simulink model "Unity_6DOFMICO_Inversekine_v8"  (R2019b)
settings: Solver=ode5  StartTime=0.0  StopTime=inf  FixedStep=0.001  RelTol=1e-3
undefined symbols (not defined in the file): f, Sub02MIHM
libraries: instrumentlib x10, simulink x10, dspnetwork x6, powerlib_meascontrol x3, dspsrcs4 x1
(part 1 of 3)
settings Model: Creator=nisit  LastModifiedBy=e295q643

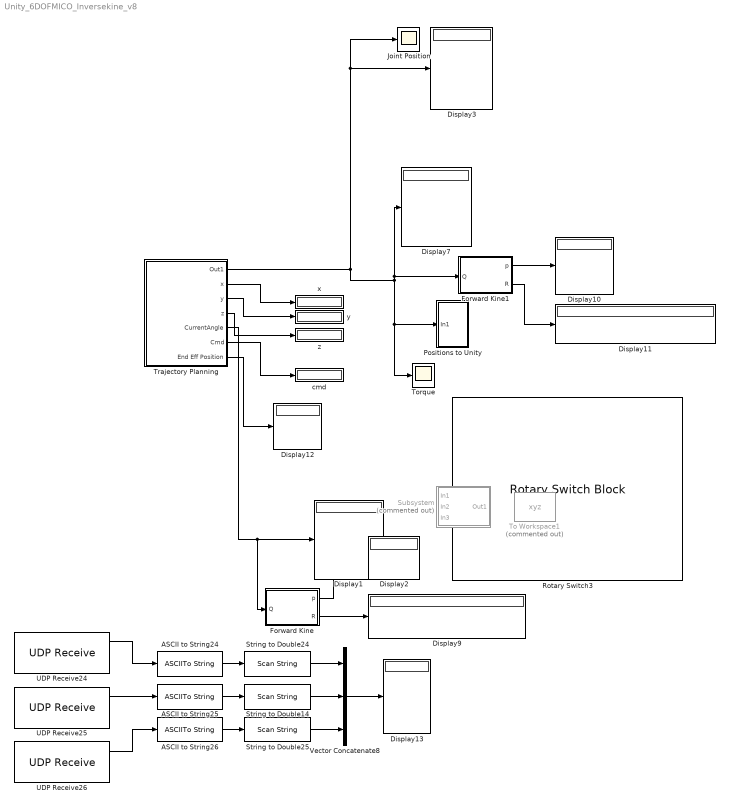
== system Unity_6DOFMICO_Inversekine_v8 ==
  ASCII to String24 : ASCIIToString
  ASCII to String25 : ASCIIToString
  ASCII to String26 : ASCIIToString
  Display{1..3,7,9..13} (9 alike) : Display
  Forward Kine : MATLAB Function  TreatAsAtomicUnit=on
  Forward Kine1 : MATLAB Function  TreatAsAtomicUnit=on
  Joint Position : Scope
  Positions to Unity : Subsystem
  Rotary Switch3 : RotarySwitchBlock
      settings: Values={{'Left', 'Right', 'Up', 'Down', 'In', 'Out', 'Resting', 'Reset'}, [1 2 3 4 5 6 7 8]}
  String to Double14 : ScanString  Format="\"%lf\""
  String to Double24 : ScanString  Format="\"%lf\""
  String to Double25 : ScanString  Format="\"%lf\""
  Subsystem : Subsystem  Commented=on
  To Workspace1 : ToWorkspace  Commented=on  VariableName=xyz  SampleTime=-1
      settings: Save2DSignal=2-D array (concatenate along first dimension)
  Torque : Scope
  Trajectory Planning : Subsystem
  UDP Receive24 : instrumentlib/UDP Receive  Host=localhost  Port=5100  LocalPort=5100  EnablePortSharing=off  GetLatestData=off  DataSize="[5  1]"  DataType=uint8  ASCIIFormatting=%f,  Terminator=LF  ByteOrder=BigEndian  EnableBlockingMode=off  Timeout=10  SampleTime=0.01  LocalAddress=127.0.0.1
  UDP Receive25 : instrumentlib/UDP Receive  Host=localhost  Port=5200  LocalPort=5200  EnablePortSharing=off  GetLatestData=off  DataSize="[5  1]"  DataType=uint8  ASCIIFormatting=%f,  Terminator=LF  ByteOrder=BigEndian  EnableBlockingMode=off  Timeout=10  SampleTime=0.01  LocalAddress=127.0.0.1
  UDP Receive26 : instrumentlib/UDP Receive  Host=localhost  Port=5300  LocalPort=5300  EnablePortSharing=off  GetLatestData=off  DataSize="[5  1]"  DataType=uint8  ASCIIFormatting=%f,  Terminator=LF  ByteOrder=BigEndian  EnableBlockingMode=off  Timeout=10  SampleTime=0.01  LocalAddress=127.0.0.1
  Vector Concatenate8 : Concatenate  NumInputs=3
  cmd : Display
  x : Display
  y : Display
  z : Display
  wires:
  Trajectory Planning/2(x) -> x/1
  Trajectory Planning/3(y) -> y/1
  Trajectory Planning/4(z) -> z/1
  Trajectory Planning/5("CurrentAngle ") -> Display1/1, Forward Kine/1(Q)
  Forward Kine/1(p) -> Display2/1
  Forward Kine/2(R) -> Display9/1
  Forward Kine1/2(R) -> Display11/1
  Forward Kine1/1(p) -> Display10/1
  Trajectory Planning/1(Out1) -> Display7/1, Forward Kine1/1(Q), Torque/1, Positions to Unity/1(In1), Display3/1, Joint Position/1
  Trajectory Planning/6(Cmd) -> cmd/1
  Subsystem/1(Out1) -> To Workspace1/1
  Trajectory Planning/7(End Eff Position) -> Display12/1
  Vector Concatenate8/1 -> Display13/1
  UDP Receive24/1 -> ASCII to String24/1
  String to Double24/1 -> Vector Concatenate8/1
  ASCII to String26/1 -> String to Double25/1
  UDP Receive25/1 -> ASCII to String25/1
  UDP Receive26/1 -> ASCII to String26/1
  String to Double25/1 -> Vector Concatenate8/3
  String to Double14/1 -> Vector Concatenate8/2
  ASCII to String24/1 -> String to Double24/1
  ASCII to String25/1 -> String to Double14/1

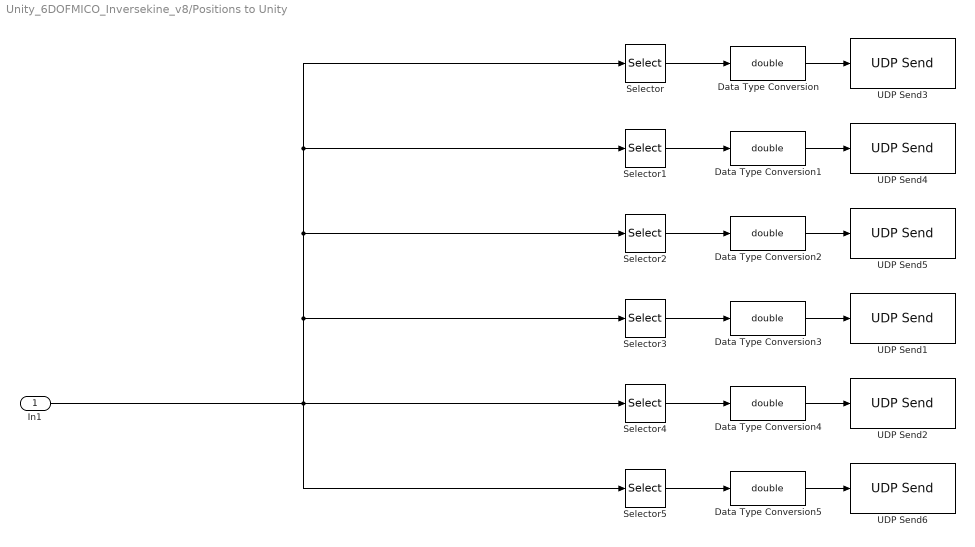
== system Unity_6DOFMICO_Inversekine_v8/Positions to Unity ==
  In1 : Inport
  Data Type Conversion{,1..5} (6 alike) : DataTypeConversion  OutDataTypeStr=double  ConvertRealWorld=Stored Integer (SI)
  Selector : Selector  InputPortWidth=6  IndexOptions=Index vector (dialog)  Indices=[1]  OutputSizes=1
  Selector1 : Selector  InputPortWidth=6  IndexOptions=Index vector (dialog)  Indices=[2]  OutputSizes=1
  Selector2 : Selector  InputPortWidth=6  IndexOptions=Index vector (dialog)  Indices=[3]  OutputSizes=1
  Selector3 : Selector  InputPortWidth=6  IndexOptions=Index vector (dialog)  Indices=[4]  OutputSizes=1
  Selector4 : Selector  InputPortWidth=6  IndexOptions=Index vector (dialog)  Indices=[5]  OutputSizes=1
  Selector5 : Selector  InputPortWidth=6  IndexOptions=Index vector (dialog)  Indices=[6]  OutputSizes=1
  UDP Send1 : dspnetwork/UDP Send  remoteURL='127.0.0.1'  remotePort=3004  localURL='0.0.0.0'  localPortSource=Automatically determine  localPort=-1  sampletime=-1  blockPlatform=[]  separateLengthPort=0
  UDP Send2 : dspnetwork/UDP Send  remoteURL='127.0.0.1'  remotePort=3005  localURL='0.0.0.0'  localPortSource=Automatically determine  localPort=-1  sampletime=-1  blockPlatform=[]  separateLengthPort=0
  UDP Send3 : dspnetwork/UDP Send  remoteURL='127.0.0.1'  remotePort=3001  localURL='0.0.0.0'  localPortSource=Automatically determine  localPort=-1  sampletime=-1  blockPlatform=[]  separateLengthPort=0
  UDP Send4 : dspnetwork/UDP Send  remoteURL='127.0.0.1'  remotePort=3002  localURL='0.0.0.0'  localPortSource=Automatically determine  localPort=-1  sampletime=-1  blockPlatform=[]  separateLengthPort=0
  UDP Send5 : dspnetwork/UDP Send  remoteURL='127.0.0.1'  remotePort=3003  localURL='0.0.0.0'  localPortSource=Automatically determine  localPort=-1  sampletime=-1  blockPlatform=[]  separateLengthPort=0
  UDP Send6 : dspnetwork/UDP Send  remoteURL='127.0.0.1'  remotePort=3006  localURL='0.0.0.0'  localPortSource=Automatically determine  localPort=-1  sampletime=-1  blockPlatform=[]  separateLengthPort=0
  wires:
  Data Type Conversion2/1 -> UDP Send5/1
  Selector5/1 -> Data Type Conversion5/1
  In1/1 -> Selector/1, Selector1/1, Selector2/1, Selector3/1, Selector5/1, Selector4/1
  Selector2/1 -> Data Type Conversion2/1
  Data Type Conversion3/1 -> UDP Send1/1
  Data Type Conversion1/1 -> UDP Send4/1
  Data Type Conversion5/1 -> UDP Send6/1
  Selector1/1 -> Data Type Conversion1/1
  Selector4/1 -> Data Type Conversion4/1
  Selector3/1 -> Data Type Conversion3/1
  Data Type Conversion4/1 -> UDP Send2/1
  Selector/1 -> Data Type Conversion/1
  Data Type Conversion/1 -> UDP Send3/1

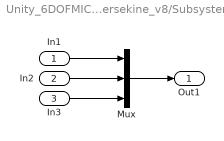
== system Unity_6DOFMICO_Inversekine_v8/Subsystem ==
  In1 : Inport
  In2 : Inport  Port=2
  In3 : Inport  Port=3
  Mux : Mux  Inputs=3
  Out1 : Outport
  wires:
  In1/1 -> Mux/1
  In2/1 -> Mux/2
  Mux/1 -> Out1/1
  In3/1 -> Mux/3

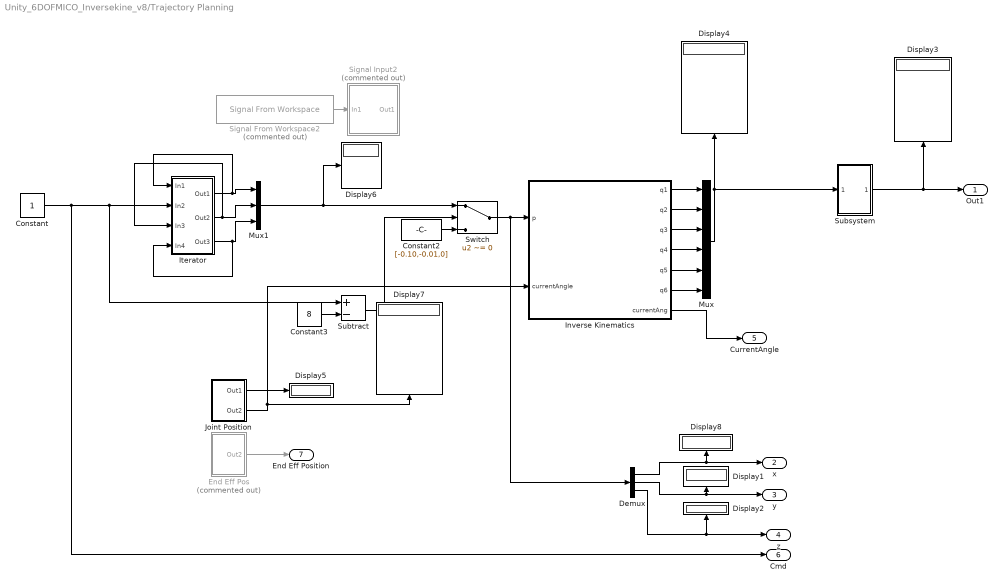
== system Unity_6DOFMICO_Inversekine_v8/Trajectory Planning ==
  Constant : Constant
  Constant2 : Constant  Value=[-0.10,-0.01,0]
  Constant3 : Constant  Value=8
  Demux : Demux  Outputs=3
  Display{1..8} (8 alike) : Display
  End Eff Pos : Subsystem  Commented=on
  Inverse Kinematics : MATLAB Function  TreatAsAtomicUnit=on
  Iterator : Subsystem
  Joint Position : Subsystem
  Mux : Mux  Inputs=6
      settings: DisplayOption=signals
  Mux1 : Mux  Inputs=3
  Signal From Workspace2 : dspsrcs4/Signal From Workspace  Commented=on  X=transpose(Sub02MIHM)  Ts=0.004  nsamps=1  OutputAfterFinalValue=Setting to zero  ignoreOrWarnInputAndFrameLengths=off  OutputFrames=off
  Signal Input2 : Subsystem  Commented=on
  Subsystem : Subsystem
  Subtract : Sum  Inputs=+-
  Switch : Switch  Criteria=u2 ~= 0
  Out1 : Outport
  x : Outport  Port=2
  y : Outport  Port=3
  z : Outport  Port=4
  "CurrentAngle " : Outport  Port=5
  Cmd : Outport  Port=6
  End Eff Position : Outport  Port=7
  wires:
  Iterator/2(Out2) -> Mux1/2, Iterator/3(In3)
  Iterator/1(Out1) -> Mux1/1, Iterator/1(In1)
  Inverse Kinematics/2(q2) -> Mux/2
  Iterator/3(Out3) -> Mux1/3, Iterator/4(In4)
  Inverse Kinematics/6(q6) -> Mux/6
  Inverse Kinematics/4(q4) -> Mux/4
  Inverse Kinematics/1(q1) -> Mux/1
  Inverse Kinematics/3(q3) -> Mux/3
  Signal From Workspace2/1 -> Signal Input2/1(In1)
  Mux/1 -> Subsystem/1(In1), Display4/1
  Inverse Kinematics/5(q5) -> Mux/5
  Subsystem/1(Out1) -> Out1/1, Display3/1
  Joint Position/1(Out1) -> Display5/1
  Joint Position/2(Out2) -> Display7/1, Inverse Kinematics/2(currentAngle)
  Demux/1 -> Display8/1, x/1
  Demux/2 -> Display1/1, y/1
  Demux/3 -> Display2/1, z/1
  Mux1/1 -> Display6/1, Switch/1
  Subtract/1 -> Switch/2
  Constant2/1 -> Switch/3
  Constant3/1 -> Subtract/2
  Constant/1 -> Cmd/1, Subtract/1, Iterator/2(In2)
  Switch/1 -> Demux/1, Inverse Kinematics/1(p)
  Inverse Kinematics/7(currentAng) -> "CurrentAngle "/1
  End Eff Pos/1(Out2) -> End Eff Position/1

== system Unity_6DOFMICO_Inversekine_v8/Trajectory Planning/End Eff Pos ==
  ASCII to String : ASCIIToString
  Display : Display
  String to Double : ScanString  Format="\"%lf\""
  UDP Receive : instrumentlib/UDP Receive  Host=localhost  Port=5000  LocalPort=5000  EnablePortSharing=off  GetLatestData=off  DataSize="[3  1]"  DataType=uint8  ASCIIFormatting=%f,  Terminator=LF  ByteOrder=BigEndian  EnableBlockingMode=off  Timeout=10  SampleTime=0.01  LocalAddress=127.0.0.1
  Out2 : Outport
  wires:
  UDP Receive/2 -> Display/1
  ASCII to String/1 -> String to Double/1
  UDP Receive/1 -> ASCII to String/1
  String to Double/1 -> Out2/1

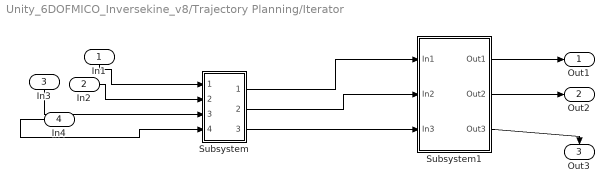
== system Unity_6DOFMICO_Inversekine_v8/Trajectory Planning/Iterator ==
  In1 : Inport
  In2 : Inport  Port=2
  In3 : Inport  Port=3
  In4 : Inport  Port=4
  Subsystem : Subsystem
  Subsystem1 : Subsystem  VariantControlMode=Label  Variant=on  VariantControl=Variant1  LabelModeActiveChoice=Variant1
  Out1 : Outport
  Out2 : Outport  Port=2
  Out3 : Outport  Port=3
  wires:
  In1/1 -> Subsystem/1(In1)
  In3/1 -> Subsystem/3(In3)
  In4/1 -> Subsystem/4(In4)
  In2/1 -> Subsystem/2(In2)
  Subsystem/1(Out1) -> Subsystem1/1("In1 ")
  Subsystem/2(Out2) -> Subsystem1/2("In2 ")
  Subsystem/3(Out3) -> Subsystem1/3("In3 ")
  Subsystem1/1(" Out1") -> Out1/1
  Subsystem1/2(" Out2") -> Out2/1
  Subsystem1/3(" Out3") -> Out3/1

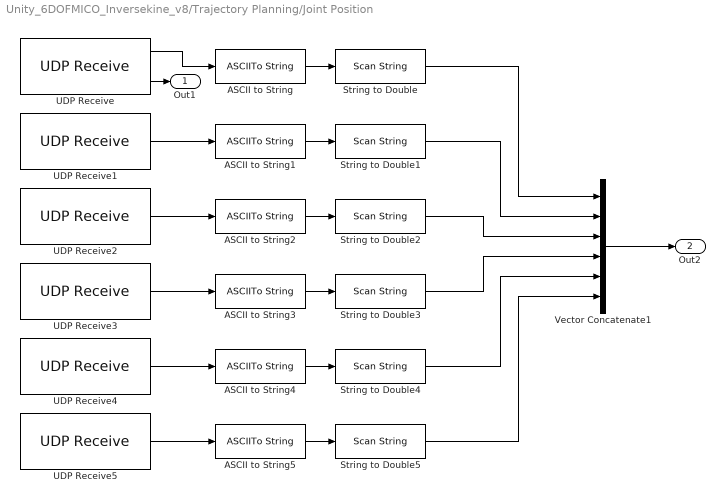
== system Unity_6DOFMICO_Inversekine_v8/Trajectory Planning/Joint Position ==
  ASCII to String{,1..5} (6 alike) : ASCIIToString
  String to Double{,1..5} (6 alike) : ScanString  Format="\"%lf\""
  UDP Receive : instrumentlib/UDP Receive  Host=localhost  Port=2001  LocalPort=2001  EnablePortSharing=off  GetLatestData=off  DataSize="[5  1]"  DataType=uint8  ASCIIFormatting=%f,  Terminator=LF  ByteOrder=BigEndian  EnableBlockingMode=off  Timeout=10  SampleTime=0.01  LocalAddress=127.0.0.1
  UDP Receive1 : instrumentlib/UDP Receive  Host=localhost  Port=2002  LocalPort=2002  EnablePortSharing=off  GetLatestData=off  DataSize="[5  1]"  DataType=uint8  ASCIIFormatting=%f,  Terminator=LF  ByteOrder=BigEndian  EnableBlockingMode=on  Timeout=10  SampleTime=0.01  LocalAddress=127.0.0.1
  UDP Receive2 : instrumentlib/UDP Receive  Host=localhost  Port=2003  LocalPort=2003  EnablePortSharing=off  GetLatestData=off  DataSize="[5  1]"  DataType=uint8  ASCIIFormatting=%f,  Terminator=LF  ByteOrder=BigEndian  EnableBlockingMode=on  Timeout=10  SampleTime=0.01  LocalAddress=127.0.0.1
  UDP Receive3 : instrumentlib/UDP Receive  Host=localhost  Port=2004  LocalPort=2004  EnablePortSharing=off  GetLatestData=off  DataSize="[5  1]"  DataType=uint8  ASCIIFormatting=%f,  Terminator=LF  ByteOrder=BigEndian  EnableBlockingMode=on  Timeout=10  SampleTime=0.01  LocalAddress=127.0.0.1
  UDP Receive4 : instrumentlib/UDP Receive  Host=localhost  Port=2005  LocalPort=2005  EnablePortSharing=off  GetLatestData=off  DataSize="[5  1]"  DataType=uint8  ASCIIFormatting=%f,  Terminator=LF  ByteOrder=BigEndian  EnableBlockingMode=on  Timeout=10  SampleTime=0.01  LocalAddress=127.0.0.1
  UDP Receive5 : instrumentlib/UDP Receive  Host=localhost  Port=2006  LocalPort=2006  EnablePortSharing=off  GetLatestData=off  DataSize="[5  1]"  DataType=uint8  ASCIIFormatting=%f,  Terminator=LF  ByteOrder=BigEndian  EnableBlockingMode=on  Timeout=10  SampleTime=0.01  LocalAddress=127.0.0.1
  Vector Concatenate1 : Concatenate  NumInputs=6
  Out1 : Outport
  Out2 : Outport  Port=2
  wires:
  String to Double3/1 -> Vector Concatenate1/4
  String to Double4/1 -> Vector Concatenate1/5
  UDP Receive1/1 -> ASCII to String1/1
  String to Double1/1 -> Vector Concatenate1/2
  UDP Receive4/1 -> ASCII to String4/1
  UDP Receive3/1 -> ASCII to String3/1
  String to Double/1 -> Vector Concatenate1/1
  ASCII to String4/1 -> String to Double4/1
  String to Double2/1 -> Vector Concatenate1/3
  ASCII to String2/1 -> String to Double2/1
  ASCII to String3/1 -> String to Double3/1
  Vector Concatenate1/1 -> Out2/1
  String to Double5/1 -> Vector Concatenate1/6
  ASCII to String1/1 -> String to Double1/1
  UDP Receive/1 -> ASCII to String/1
  UDP Receive5/1 -> ASCII to String5/1
  UDP Receive2/1 -> ASCII to String2/1
  ASCII to String5/1 -> String to Double5/1
  ASCII to String/1 -> String to Double/1
  UDP Receive/2 -> Out1/1

== system Unity_6DOFMICO_Inversekine_v8/Trajectory Planning/Signal Input2 ==
  In1 : Inport
  Iterator Input : Subsystem
  Subsystem1 : Subsystem
  Out1 : Outport
  wires:
  Subsystem1/1(Out1) -> Iterator Input/1(In1)
  Subsystem1/3(Out3) -> Iterator Input/3(In3)
  In1/1 -> Subsystem1/1(In1)
  Subsystem1/4(Out4) -> Iterator Input/4(In4)
  Subsystem1/7(Out7) -> Iterator Input/7(In7)
  Subsystem1/2(Out2) -> Iterator Input/2(In2)
  Subsystem1/6(Out6) -> Iterator Input/6(In6)
  Subsystem1/5(Out5) -> Iterator Input/5(In5)
  Iterator Input/1(Out1) -> Out1/1

== system Unity_6DOFMICO_Inversekine_v8/Trajectory Planning/Subsystem ==
  In1 : Inport
  Demux : Demux  Outputs=6
  Mux1 : Mux  Inputs=6
  Out1 : Outport
  wires:
  Demux/2 -> Mux1/2
  Demux/5 -> Mux1/5
  Demux/1 -> Mux1/1
  Mux1/1 -> Out1/1
  Demux/6 -> Mux1/6
  In1/1 -> Demux/1
  Demux/4 -> Mux1/4
  Demux/3 -> Mux1/3

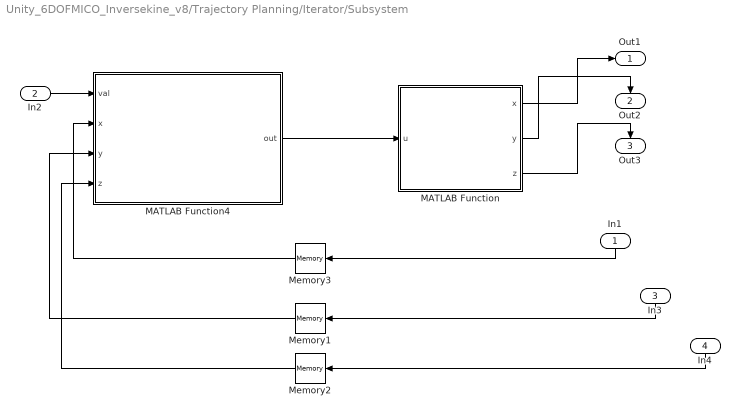
== system Unity_6DOFMICO_Inversekine_v8/Trajectory Planning/Iterator/Subsystem ==
  In1 : Inport
  In2 : Inport  Port=2
  In3 : Inport  Port=3
  In4 : Inport  Port=4
  MATLAB Function : MATLAB Function  TreatAsAtomicUnit=on
  MATLAB Function4 : MATLAB Function  TreatAsAtomicUnit=on
  Memory1 : Memory
  Memory2 : Memory
  Memory3 : Memory
  Out1 : Outport
  Out2 : Outport  Port=2
  Out3 : Outport  Port=3
  wires:
  In2/1 -> MATLAB Function4/1(val)
  MATLAB Function/2(y) -> Out2/1
  MATLAB Function/3(z) -> Out3/1
  MATLAB Function/1(x) -> Out1/1
  MATLAB Function4/1(out) -> MATLAB Function/1(u)
  In1/1 -> Memory3/1
  In3/1 -> Memory1/1
  In4/1 -> Memory2/1
  Memory3/1 -> MATLAB Function4/2(x)
  Memory1/1 -> MATLAB Function4/3(y)
  Memory2/1 -> MATLAB Function4/4(z)

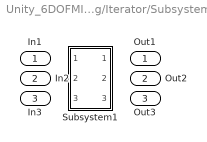
== system Unity_6DOFMICO_Inversekine_v8/Trajectory Planning/Iterator/Subsystem1 ==
  "In1 " : Inport
  "In2 " : Inport  Port=2
  "In3 " : Inport  Port=3
  Subsystem1 : Subsystem  VariantControl=Variant1
  " Out1" : Outport
  " Out2" : Outport  Port=2
  " Out3" : Outport  Port=3

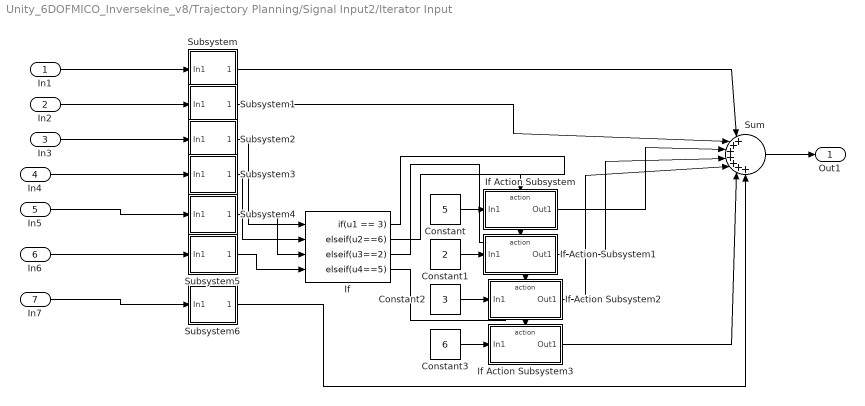
== system Unity_6DOFMICO_Inversekine_v8/Trajectory Planning/Signal Input2/Iterator Input ==
  In1 : Inport
  In2 : Inport  Port=2
  In3 : Inport  Port=3
  In4 : Inport  Port=4
  In5 : Inport  Port=5
  In6 : Inport  Port=6
  In7 : Inport  Port=7
  Constant : Constant  Value=5
  Constant1 : Constant  Value=2
  Constant2 : Constant  Value=3
  Constant3 : Constant  Value=6
  If : If  NumInputs=4  IfExpression=u1 == 3  ElseIfExpressions=u2==6,u3==2,u4==5  ShowElse=off
  If Action Subsystem : Subsystem  TreatAsAtomicUnit=on
  If Action Subsystem1 : Subsystem  TreatAsAtomicUnit=on
  If Action Subsystem2 : Subsystem  TreatAsAtomicUnit=on
  If Action Subsystem3 : Subsystem  TreatAsAtomicUnit=on
  Subsystem : Subsystem
  Subsystem1 : Subsystem
  Subsystem2 : Subsystem
  Subsystem3 : Subsystem
  Subsystem4 : Subsystem
  Subsystem5 : Subsystem
  Subsystem6 : Subsystem
  Sum : Sum  Inputs=|+++++++
  Out1 : Outport
  wires:
  Sum/1 -> Out1/1
  In5/1 -> Subsystem4/1(In1)
  In2/1 -> Subsystem1/1(In1)
  Subsystem/1(Out1) -> Sum/1
  In4/1 -> Subsystem3/1(In1)
  Subsystem1/1(Out1) -> Sum/2
  In1/1 -> Subsystem/1(In1)
  In3/1 -> Subsystem2/1(In1)
  In6/1 -> Subsystem5/1(In1)
  In7/1 -> Subsystem6/1(In1)
  If/1 -> If Action Subsystem/Action
  Constant/1 -> If Action Subsystem/1(In1)
  If/2 -> If Action Subsystem1/Action
  If/3 -> If Action Subsystem2/Action
  If/4 -> If Action Subsystem3/Action
  Constant2/1 -> If Action Subsystem2/1(In1)
  Constant1/1 -> If Action Subsystem1/1(In1)
  Constant3/1 -> If Action Subsystem3/1(In1)
  Subsystem2/1(Out1) -> If/1
  Subsystem3/1(Out1) -> If/2
  Subsystem4/1(Out1) -> If/3
  Subsystem5/1(Out1) -> If/4
  Subsystem6/1(Out1) -> Sum/7
  If Action Subsystem/1(Out1) -> Sum/3
  If Action Subsystem1/1(Out1) -> Sum/4
  If Action Subsystem2/1(Out1) -> Sum/5
  If Action Subsystem3/1(Out1) -> Sum/6

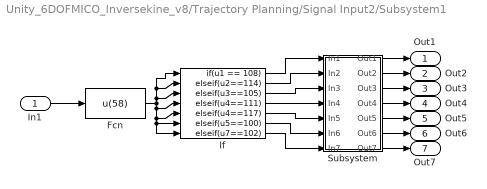
== system Unity_6DOFMICO_Inversekine_v8/Trajectory Planning/Signal Input2/Subsystem1 ==
  In1 : Inport
  Fcn : Fcn  Expr=u(58)
  If : If  NumInputs=7  IfExpression=u1 == 108  ElseIfExpressions=u2==114,u3==105,u4==111,u4==117,u5==100,u7==102  ShowElse=off
  Subsystem : Subsystem
  Out1 : Outport
  Out2 : Outport  Port=2
  Out3 : Outport  Port=3
  Out4 : Outport  Port=4
  Out5 : Outport  Port=5
  Out6 : Outport  Port=6
  Out7 : Outport  Port=7
  wires:
  If/6 -> Subsystem/6(In6)
  If/2 -> Subsystem/2(In2)
  If/4 -> Subsystem/4(In4)
  If/7 -> Subsystem/7(In7)
  If/3 -> Subsystem/3(In3)
  Fcn/1 -> If/1, If/2, If/3, If/7, If/6, If/5, If/4
  If/1 -> Subsystem/1(In1)
  If/5 -> Subsystem/5(In5)
  Subsystem/1(Out1) -> Out1/1
  Subsystem/2(Out2) -> Out2/1
  Subsystem/3(Out3) -> Out3/1
  In1/1 -> Fcn/1
  Subsystem/6(Out6) -> Out6/1
  Subsystem/5(Out5) -> Out5/1
  Subsystem/4(Out4) -> Out4/1
  Subsystem/7(Out7) -> Out7/1

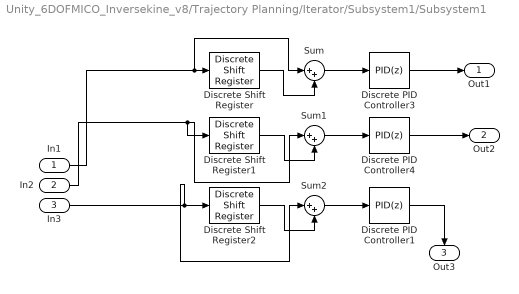
== system Unity_6DOFMICO_Inversekine_v8/Trajectory Planning/Iterator/Subsystem1/Subsystem1 ==
  In1 : Inport
  In2 : Inport  Port=2
  In3 : Inport  Port=3
  Discrete Shift Register : powerlib_meascontrol/Additional Components/Discrete Shift Register  NSamples=1  InitialValue=0  Ts=-1
      settings: SourceProductName=Simscape Electrical  SourceProductBaseCode=PS
  Discrete Shift Register1 : powerlib_meascontrol/Additional Components/Discrete Shift Register  NSamples=1  InitialValue=0  Ts=-1
      settings: SourceProductName=Simscape Electrical  SourceProductBaseCode=PS
  Discrete Shift Register2 : powerlib_meascontrol/Additional Components/Discrete Shift Register  NSamples=1  InitialValue=0  Ts=-1
      settings: SourceProductName=Simscape Electrical  SourceProductBaseCode=PS
  Discrete PID Controller1 : simulink/Continuous/PID Controller  Controller=PID  Form=Parallel  TimeDomain=Discrete-time  SampleTime=-1  IntegratorMethod=Forward Euler  FilterMethod=Forward Euler  ControllerParametersSource=internal  P=1  I=1  D=0  UseFilter=on  N=100  TunerSelectOption=Transfer Function Based (PID Tuner App)  InitialConditionSource=internal  InitialConditionForIntegrator=0  InitialConditionForFilter=0  DifferentiatorICPrevScaledInput=0  ExternalReset=none  TrackingMode=off  Kt=1  LimitOutput=off  UpperSaturationLimit=inf  LowerSaturationLimit=-inf  LinearizeAsGain=off  AntiWindupMode=none  Kb=1  POutMin=[]  POutMax=[]  IOutMin=[]  IOutMax=[]  DOutMin=[]  DOutMax=[]  NOutMin=[]  NOutMax=[]  SumOutMin=[]  SumOutMax=[]  SaturationOutMin=[]  SaturationOutMax=[]  PParamMin=[]  PParamMax=[]  IParamMin=[]  IParamMax=[]  DParamMin=[]  DParamMax=[]  NParamMin=[]  NParamMax=[]  KbParamMin=[]  KbParamMax=[]  KtParamMin=[]  KtParamMax=[]  KbOutMin=[]  KbOutMax=[]  KtOutMin=[]  KtOutMax=[]  IntegratorOutMin=[]  IntegratorOutMax=[]  FilterOutMin=[]  FilterOutMax=[]  SumI1OutMin=[]  SumI1OutMax=[]  SumI2OutMin=[]  SumI2OutMax=[]  SumI3OutMin=[]  SumI3OutMax=[]  SumI4OutMin=[]  SumI4OutMax=[]  SumDOutMin=[]  SumDOutMax=[]  DifferentiatorOutMin=[]  DifferentiatorOutMax=[]  FilterDiffOutCoefMin=[]  FilterDiffOutCoefMax=[]  ReciprocalOutMin=[]  ReciprocalOutMax=[]  SumDenOutMin=[]  SumDenOutMax=[]  SumNumOutMin=[]  SumNumOutMax=[]  DivideOutMin=[]  DivideOutMax=[]  IntegratorContinuousStateAttributes=''  IntegratorStateMustResolveToSignalObject=off  IntegratorRTWStateStorageClass=Auto  FilterContinuousStateAttributes=''  FilterStateMustResolveToSignalObject=off  FilterRTWStateStorageClass=Auto  ParallelPVariant=InternalParameters  IdealPVariant=Disabled  IVariant=InternalParameters  DVariant=InternalParameters  IntegratorVariant=Discrete  SatVariant=Disabled  AWVariant=Passthrough  PCopyVariant=Disabled  TRVariant=Disabled  FdbkBlocksVariant=Forward  IdealPFdbkVariant=Disabled  SatFdbkVariant=Disabled  DerivativeFilterVariant=ForwardEulerFilter  NVariant=InternalParameters  NCopyVariant=Disabled  FilterICVariant=InternalICsFilter  IntegratorICVariant=InternalICs  ExternalResetVariant=Disabled  TRSumVariant=Passthrough  SumFdbkVariant=Disabled  SumVariant=Sum_PID
  Discrete PID Controller3 : simulink/Continuous/PID Controller  Controller=PID  Form=Parallel  TimeDomain=Discrete-time  SampleTime=-1  IntegratorMethod=Forward Euler  FilterMethod=Forward Euler  ControllerParametersSource=internal  P=1  I=1  D=0  UseFilter=on  N=100  TunerSelectOption=Transfer Function Based (PID Tuner App)  InitialConditionSource=internal  InitialConditionForIntegrator=0  InitialConditionForFilter=0  DifferentiatorICPrevScaledInput=0  ExternalReset=none  TrackingMode=off  Kt=1  LimitOutput=off  UpperSaturationLimit=inf  LowerSaturationLimit=-inf  LinearizeAsGain=off  AntiWindupMode=none  Kb=1  POutMin=[]  POutMax=[]  IOutMin=[]  IOutMax=[]  DOutMin=[]  DOutMax=[]  NOutMin=[]  NOutMax=[]  SumOutMin=[]  SumOutMax=[]  SaturationOutMin=[]  SaturationOutMax=[]  PParamMin=[]  PParamMax=[]  IParamMin=[]  IParamMax=[]  DParamMin=[]  DParamMax=[]  NParamMin=[]  NParamMax=[]  KbParamMin=[]  KbParamMax=[]  KtParamMin=[]  KtParamMax=[]  KbOutMin=[]  KbOutMax=[]  KtOutMin=[]  KtOutMax=[]  IntegratorOutMin=[]  IntegratorOutMax=[]  FilterOutMin=[]  FilterOutMax=[]  SumI1OutMin=[]  SumI1OutMax=[]  SumI2OutMin=[]  SumI2OutMax=[]  SumI3OutMin=[]  SumI3OutMax=[]  SumI4OutMin=[]  SumI4OutMax=[]  SumDOutMin=[]  SumDOutMax=[]  DifferentiatorOutMin=[]  DifferentiatorOutMax=[]  FilterDiffOutCoefMin=[]  FilterDiffOutCoefMax=[]  ReciprocalOutMin=[]  ReciprocalOutMax=[]  SumDenOutMin=[]  SumDenOutMax=[]  SumNumOutMin=[]  SumNumOutMax=[]  DivideOutMin=[]  DivideOutMax=[]  IntegratorContinuousStateAttributes=''  IntegratorStateMustResolveToSignalObject=off  IntegratorRTWStateStorageClass=Auto  FilterContinuousStateAttributes=''  FilterStateMustResolveToSignalObject=off  FilterRTWStateStorageClass=Auto  ParallelPVariant=InternalParameters  IdealPVariant=Disabled  IVariant=InternalParameters  DVariant=InternalParameters  IntegratorVariant=Discrete  SatVariant=Disabled  AWVariant=Passthrough  PCopyVariant=Disabled  TRVariant=Disabled  FdbkBlocksVariant=Forward  IdealPFdbkVariant=Disabled  SatFdbkVariant=Disabled  DerivativeFilterVariant=ForwardEulerFilter  NVariant=InternalParameters  NCopyVariant=Disabled  FilterICVariant=InternalICsFilter  IntegratorICVariant=InternalICs  ExternalResetVariant=Disabled  TRSumVariant=Passthrough  SumFdbkVariant=Disabled  SumVariant=Sum_PID
  Discrete PID Controller4 : simulink/Continuous/PID Controller  Controller=PID  Form=Parallel  TimeDomain=Discrete-time  SampleTime=-1  IntegratorMethod=Forward Euler  FilterMethod=Forward Euler  ControllerParametersSource=internal  P=1  I=1  D=0  UseFilter=on  N=100  TunerSelectOption=Transfer Function Based (PID Tuner App)  InitialConditionSource=internal  InitialConditionForIntegrator=0  InitialConditionForFilter=0  DifferentiatorICPrevScaledInput=0  ExternalReset=none  TrackingMode=off  Kt=1  LimitOutput=off  UpperSaturationLimit=inf  LowerSaturationLimit=-inf  LinearizeAsGain=off  AntiWindupMode=none  Kb=1  POutMin=[]  POutMax=[]  IOutMin=[]  IOutMax=[]  DOutMin=[]  DOutMax=[]  NOutMin=[]  NOutMax=[]  SumOutMin=[]  SumOutMax=[]  SaturationOutMin=[]  SaturationOutMax=[]  PParamMin=[]  PParamMax=[]  IParamMin=[]  IParamMax=[]  DParamMin=[]  DParamMax=[]  NParamMin=[]  NParamMax=[]  KbParamMin=[]  KbParamMax=[]  KtParamMin=[]  KtParamMax=[]  KbOutMin=[]  KbOutMax=[]  KtOutMin=[]  KtOutMax=[]  IntegratorOutMin=[]  IntegratorOutMax=[]  FilterOutMin=[]  FilterOutMax=[]  SumI1OutMin=[]  SumI1OutMax=[]  SumI2OutMin=[]  SumI2OutMax=[]  SumI3OutMin=[]  SumI3OutMax=[]  SumI4OutMin=[]  SumI4OutMax=[]  SumDOutMin=[]  SumDOutMax=[]  DifferentiatorOutMin=[]  DifferentiatorOutMax=[]  FilterDiffOutCoefMin=[]  FilterDiffOutCoefMax=[]  ReciprocalOutMin=[]  ReciprocalOutMax=[]  SumDenOutMin=[]  SumDenOutMax=[]  SumNumOutMin=[]  SumNumOutMax=[]  DivideOutMin=[]  DivideOutMax=[]  IntegratorContinuousStateAttributes=''  IntegratorStateMustResolveToSignalObject=off  IntegratorRTWStateStorageClass=Auto  FilterContinuousStateAttributes=''  FilterStateMustResolveToSignalObject=off  FilterRTWStateStorageClass=Auto  ParallelPVariant=InternalParameters  IdealPVariant=Disabled  IVariant=InternalParameters  DVariant=InternalParameters  IntegratorVariant=Discrete  SatVariant=Disabled  AWVariant=Passthrough  PCopyVariant=Disabled  TRVariant=Disabled  FdbkBlocksVariant=Forward  IdealPFdbkVariant=Disabled  SatFdbkVariant=Disabled  DerivativeFilterVariant=ForwardEulerFilter  NVariant=InternalParameters  NCopyVariant=Disabled  FilterICVariant=InternalICsFilter  IntegratorICVariant=InternalICs  ExternalResetVariant=Disabled  TRSumVariant=Passthrough  SumFdbkVariant=Disabled  SumVariant=Sum_PID
  Sum : Sum  Inputs=|++
  Sum1 : Sum  Inputs=|++
  Sum2 : Sum  Inputs=|++
  Out1 : Outport
  Out2 : Outport  Port=2
  Out3 : Outport  Port=3
  wires:
  Sum/1 -> Discrete PID Controller3/1
  Sum2/1 -> Discrete PID Controller1/1
  Sum1/1 -> Discrete PID Controller4/1
  Discrete Shift Register/1 -> Sum/2
  Discrete Shift Register1/1 -> Sum1/2
  Discrete Shift Register2/1 -> Sum2/2
  In3/1 -> Sum2/1, Discrete Shift Register2/1
  In2/1 -> Sum1/1, Discrete Shift Register1/1
  In1/1 -> Sum/1, Discrete Shift Register/1
  Discrete PID Controller1/1 -> Out3/1
  Discrete PID Controller4/1 -> Out2/1
  Discrete PID Controller3/1 -> Out1/1

== system Unity_6DOFMICO_Inversekine_v8/Trajectory Planning/Signal Input2/Iterator Input/If Action Subsystem ==
  In1 : Inport
  Action Port : ActionPort  InitializeStates=reset
  Out1 : Outport  OutputWhenDisabled=reset  InitialOutput=[0]
  wires:
  In1/1 -> Out1/1

== system Unity_6DOFMICO_Inversekine_v8/Trajectory Planning/Signal Input2/Iterator Input/If Action Subsystem1 ==
  In1 : Inport
  Action Port : ActionPort  InitializeStates=reset
  Out1 : Outport  OutputWhenDisabled=reset  InitialOutput=[0]
  wires:
  In1/1 -> Out1/1

== system Unity_6DOFMICO_Inversekine_v8/Trajectory Planning/Signal Input2/Iterator Input/If Action Subsystem2 ==
  In1 : Inport
  Action Port : ActionPort  InitializeStates=reset
  Out1 : Outport  OutputWhenDisabled=reset  InitialOutput=[0]
  wires:
  In1/1 -> Out1/1

== system Unity_6DOFMICO_Inversekine_v8/Trajectory Planning/Signal Input2/Iterator Input/If Action Subsystem3 ==
  In1 : Inport
  Action Port : ActionPort  InitializeStates=reset
  Out1 : Outport  OutputWhenDisabled=reset  InitialOutput=[0]
  wires:
  In1/1 -> Out1/1

== system Unity_6DOFMICO_Inversekine_v8/Trajectory Planning/Signal Input2/Iterator Input/Subsystem ==
  In1 : Inport
  Compare To Constant : simulink/Logic and Bit Operations/Compare To Constant  relop===  const=1  OutDataTypeStr=boolean
  Constant : Constant
  Product : Product
  Out1 : Outport
  wires:
  Constant/1 -> Product/1
  Compare To Constant/1 -> Product/2
  In1/1 -> Compare To Constant/1
  Product/1 -> Out1/1

== system Unity_6DOFMICO_Inversekine_v8/Trajectory Planning/Signal Input2/Iterator Input/Subsystem1 ==
  In1 : Inport
  Compare To Constant : simulink/Logic and Bit Operations/Compare To Constant  relop===  const=4  OutDataTypeStr=boolean
  Constant : Constant  Value=4
  Product : Product
  Out1 : Outport
  wires:
  Product/1 -> Out1/1
  In1/1 -> Compare To Constant/1
  Compare To Constant/1 -> Product/2
  Constant/1 -> Product/1

== system Unity_6DOFMICO_Inversekine_v8/Trajectory Planning/Signal Input2/Iterator Input/Subsystem2 ==
  In1 : Inport
  Compare To Constant : simulink/Logic and Bit Operations/Compare To Constant  relop===  const=3  OutDataTypeStr=boolean
  Constant : Constant  Value=3
  Product : Product
  Out1 : Outport
  wires:
  Constant/1 -> Product/1
  Compare To Constant/1 -> Product/2
  In1/1 -> Compare To Constant/1
  Product/1 -> Out1/1

== system Unity_6DOFMICO_Inversekine_v8/Trajectory Planning/Signal Input2/Iterator Input/Subsystem3 ==
  In1 : Inport
  Compare To Constant : simulink/Logic and Bit Operations/Compare To Constant  relop===  const=6  OutDataTypeStr=boolean
  Constant : Constant  Value=6
  Product : Product
  Out1 : Outport
  wires:
  Product/1 -> Out1/1
  In1/1 -> Compare To Constant/1
  Compare To Constant/1 -> Product/2
  Constant/1 -> Product/1

== system Unity_6DOFMICO_Inversekine_v8/Trajectory Planning/Signal Input2/Iterator Input/Subsystem4 ==
  In1 : Inport
  Compare To Constant : simulink/Logic and Bit Operations/Compare To Constant  relop===  const=2  OutDataTypeStr=boolean
  Constant : Constant  Value=2
  Product : Product
  Out1 : Outport
  wires:
  Constant/1 -> Product/1
  Compare To Constant/1 -> Product/2
  In1/1 -> Compare To Constant/1
  Product/1 -> Out1/1

== system Unity_6DOFMICO_Inversekine_v8/Trajectory Planning/Signal Input2/Iterator Input/Subsystem5 ==
  In1 : Inport
  Compare To Constant : simulink/Logic and Bit Operations/Compare To Constant  relop===  const=5  OutDataTypeStr=boolean
  Constant : Constant  Value=5
  Product : Product
  Out1 : Outport
  wires:
  Product/1 -> Out1/1
  In1/1 -> Compare To Constant/1
  Compare To Constant/1 -> Product/2
  Constant/1 -> Product/1

== system Unity_6DOFMICO_Inversekine_v8/Trajectory Planning/Signal Input2/Iterator Input/Subsystem6 ==
  In1 : Inport
  Compare To Constant : simulink/Logic and Bit Operations/Compare To Constant  relop===  const=0  OutDataTypeStr=boolean
  Constant : Constant  Value=0
  Product : Product
  Out1 : Outport
  wires:
  Constant/1 -> Product/1
  Compare To Constant/1 -> Product/2
  In1/1 -> Compare To Constant/1
  Product/1 -> Out1/1

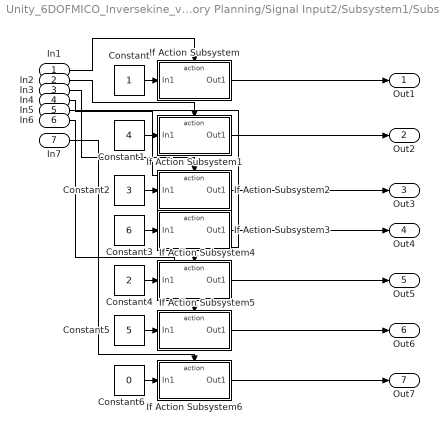
== system Unity_6DOFMICO_Inversekine_v8/Trajectory Planning/Signal Input2/Subsystem1/Subsystem ==
  In1 : Inport
  In2 : Inport  Port=2
  In3 : Inport  Port=3
  In4 : Inport  Port=4
  In5 : Inport  Port=5
  In6 : Inport  Port=6
  In7 : Inport  Port=7
  Constant : Constant
  Constant1 : Constant  Value=4
  Constant2 : Constant  Value=3
  Constant3 : Constant  Value=6
  Constant4 : Constant  Value=2
  Constant5 : Constant  Value=5
  Constant6 : Constant  Value=0
  If Action Subsystem : Subsystem  TreatAsAtomicUnit=on
  If Action Subsystem1 : Subsystem  TreatAsAtomicUnit=on
  If Action Subsystem2 : Subsystem  TreatAsAtomicUnit=on
  If Action Subsystem3 : Subsystem  TreatAsAtomicUnit=on
  If Action Subsystem4 : Subsystem  TreatAsAtomicUnit=on
  If Action Subsystem5 : Subsystem  TreatAsAtomicUnit=on
  If Action Subsystem6 : Subsystem  TreatAsAtomicUnit=on
  Out1 : Outport
  Out2 : Outport  Port=2
  Out3 : Outport  Port=3
  Out4 : Outport  Port=4
  Out5 : Outport  Port=5
  Out6 : Outport  Port=6
  Out7 : Outport  Port=7
  wires:
  Constant/1 -> If Action Subsystem/1(In1)
  In2/1 -> If Action Subsystem1/Action
  Constant2/1 -> If Action Subsystem2/1(In1)
  In4/1 -> If Action Subsystem3/Action
  Constant5/1 -> If Action Subsystem5/1(In1)
  Constant1/1 -> If Action Subsystem1/1(In1)
  In3/1 -> If Action Subsystem2/Action
  If Action Subsystem/1(Out1) -> Out1/1
  Constant3/1 -> If Action Subsystem3/1(In1)
  In1/1 -> If Action Subsystem/Action
  Constant4/1 -> If Action Subsystem4/1(In1)
  In6/1 -> If Action Subsystem5/Action
  If Action Subsystem2/1(Out1) -> Out3/1
  If Action Subsystem4/1(Out1) -> Out5/1
  If Action Subsystem3/1(Out1) -> Out4/1
  In5/1 -> If Action Subsystem4/Action
  If Action Subsystem5/1(Out1) -> Out6/1
  If Action Subsystem1/1(Out1) -> Out2/1
  Constant6/1 -> If Action Subsystem6/1(In1)
  In7/1 -> If Action Subsystem6/Action
  If Action Subsystem6/1(Out1) -> Out7/1

== system Unity_6DOFMICO_Inversekine_v8/Trajectory Planning/Signal Input2/Subsystem1/Subsystem/If Action Subsystem ==
  In1 : Inport
  Action Port : ActionPort  InitializeStates=reset
  Out1 : Outport  OutputWhenDisabled=reset  InitialOutput=[0]
  wires:
  In1/1 -> Out1/1

== system Unity_6DOFMICO_Inversekine_v8/Trajectory Planning/Signal Input2/Subsystem1/Subsystem/If Action Subsystem1 ==
  In1 : Inport
  Action Port : ActionPort  InitializeStates=reset
  Out1 : Outport  OutputWhenDisabled=reset  InitialOutput=[0]
  wires:
  In1/1 -> Out1/1

== system Unity_6DOFMICO_Inversekine_v8/Trajectory Planning/Signal Input2/Subsystem1/Subsystem/If Action Subsystem2 ==
  In1 : Inport
  Action Port : ActionPort  InitializeStates=reset
  Out1 : Outport  OutputWhenDisabled=reset  InitialOutput=[0]
  wires:
  In1/1 -> Out1/1

== system Unity_6DOFMICO_Inversekine_v8/Trajectory Planning/Signal Input2/Subsystem1/Subsystem/If Action Subsystem3 ==
  In1 : Inport
  Action Port : ActionPort  InitializeStates=reset
  Out1 : Outport  OutputWhenDisabled=reset  InitialOutput=[0]
  wires:
  In1/1 -> Out1/1

== system Unity_6DOFMICO_Inversekine_v8/Trajectory Planning/Signal Input2/Subsystem1/Subsystem/If Action Subsystem4 ==
  In1 : Inport
  Action Port : ActionPort  InitializeStates=reset
  Out1 : Outport  OutputWhenDisabled=reset  InitialOutput=[0]
  wires:
  In1/1 -> Out1/1

== system Unity_6DOFMICO_Inversekine_v8/Trajectory Planning/Signal Input2/Subsystem1/Subsystem/If Action Subsystem5 ==
  In1 : Inport
  Action Port : ActionPort  InitializeStates=reset
  Out1 : Outport  OutputWhenDisabled=reset  InitialOutput=[0]
  wires:
  In1/1 -> Out1/1

== system Unity_6DOFMICO_Inversekine_v8/Trajectory Planning/Signal Input2/Subsystem1/Subsystem/If Action Subsystem6 ==
  In1 : Inport
  Action Port : ActionPort  InitializeStates=reset
  Out1 : Outport  OutputWhenDisabled=reset  InitialOutput=[0]
  wires:
  In1/1 -> Out1/1

== matlab function Unity_6DOFMICO_Inversekine_v8/Forward Kine1 ==
  data: Q input; p output; R output
function [p,R] = fcn(Q)

%Inputs
Th_1=Q(1);
Th_2=Q(2);
Th_3=Q(3);
Th_4=Q(4);
Th_5=Q(5);
Th_6=Q(6);

% 
% Th_1=-1.6851;
% Th_2=-0.7011;
% Th_3=-3.3627;
% Th_4=0.3119;
% Th_5=1.7655;
% Th_6=-1.0709;

%DH Table
a = [0;0.4100;0;0;0;0];
b = [0.2102;0;-0.0120;-0.2493;-0.0846; -0.2273];
alpha = [90;180;90;55;55;180]*(pi/180);

% b__1 = 0.2102;  %Base to shoulder
% a__2 = 0.4100;  %Upper arm length (shoulder to elbow)
% b__3 = -0.0120; %Joint 3-4 lateral offset
% b__4 = -0.2493; %Distance from elbow to first sub-segment of the first wrist 
% %semgment
% b__5 = -0.0846; %Distance from end of the first sub-segment to of the first
% % wrist segment to end of the first sub-segment of the second wrist segment
% b__6 = -0.2273; % Distance from the end of the first sub-segment of the 
% % second wrist segment to the center of the hand.
% s__r4 = sind(55); %55 degrees is the angle of curvature first wrist segment
% s__r5 = sind(55); %55 degrees is the angle of curvature first wrist segment
% c__r4 = cosd(55); %55 degrees is the angle of curvature second wrist segment
% c__r5 = cosd(55); %55 degrees is the angle of curvature second wrist segment
% 

%Function for Transformation Matrix 
A=@(theta,a,d,alpha) ([cos(theta),-sin(theta)*cos(alpha),sin(theta)*sin(alpha),a*cos(theta);sin(theta),cos(theta)*cos(alpha),-cos(theta)*sin(alpha),a*sin(theta);0,sin(alpha),cos(alpha),d;0,0,0,1]);

% Calculate the different A matrices and then calculate the DH matrix
A1 = A(Th_1,a(1),b(1),alpha(1));
A2 = A(Th_2,a(2),b(2),alpha(2));
A3 = A(Th_3,a(3),b(3),alpha(3));
A4 = A(Th_4,a(4),b(4),alpha(4));
A5 = A(Th_5,a(5),b(5),alpha(5));
A6 = A(Th_6,a(6),b(6),alpha(6));

%Transformation Matrix 
% T1=A1;
% T2=A1*A2;
% T3=A1*A2*A3;
% T4=A1*A2*A3*A4;
% T5=A1*A2*A3*A4*A5;
T6=A1*A2*A3*A4*A5*A6;

Ox = T6(1,4);
Oy = T6(2,4);
Oz = T6(3,4);
p=[Ox;Oy;Oz]

R=T6(1:3,1:3)

== matlab function Unity_6DOFMICO_Inversekine_v8/Forward Kine ==
  data: Q input; p output; R output
function [p,R] = fcn(Q)

%Inputs
Th_1=Q(1);
Th_2=Q(2);
Th_3=Q(3);
Th_4=Q(4);
Th_5=Q(5);
Th_6=Q(6);

% 
% Th_1=-1.6851;
% Th_2=-0.7011;
% Th_3=-3.3627;
% Th_4=0.3119;
% Th_5=1.7655;
% Th_6=-1.0709;

%DH Table
a = [0;0.4100;0;0;0;0];
b = [0.2102;0;-0.0120;-0.2493;-0.0846; -0.2273];
alpha = [90;180;90;55;55;180]*(pi/180);

% b__1 = 0.2102;  %Base to shoulder
% a__2 = 0.4100;  %Upper arm length (shoulder to elbow)
% b__3 = -0.0120; %Joint 3-4 lateral offset
% b__4 = -0.2493; %Distance from elbow to first sub-segment of the first wrist 
% %semgment
% b__5 = -0.0846; %Distance from end of the first sub-segment to of the first
% % wrist segment to end of the first sub-segment of the second wrist segment
% b__6 = -0.2273; % Distance from the end of the first sub-segment of the 
% % second wrist segment to the center of the hand.
% s__r4 = sind(55); %55 degrees is the angle of curvature first wrist segment
% s__r5 = sind(55); %55 degrees is the angle of curvature first wrist segment
% c__r4 = cosd(55); %55 degrees is the angle of curvature second wrist segment
% c__r5 = cosd(55); %55 degrees is the angle of curvature second wrist segment
% 

%Function for Transformation Matrix 
A=@(theta,a,d,alpha) ([cos(theta),-sin(theta)*cos(alpha),sin(theta)*sin(alpha),a*cos(theta);sin(theta),cos(theta)*cos(alpha),-cos(theta)*sin(alpha),a*sin(theta);0,sin(alpha),cos(alpha),d;0,0,0,1]);

% Calculate the different A matrices and then calculate the DH matrix
A1 = A(Th_1,a(1),b(1),alpha(1));
A2 = A(Th_2,a(2),b(2),alpha(2));
A3 = A(Th_3,a(3),b(3),alpha(3));
A4 = A(Th_4,a(4),b(4),alpha(4));
A5 = A(Th_5,a(5),b(5),alpha(5));
A6 = A(Th_6,a(6),b(6),alpha(6));

%Transformation Matrix 
% T1=A1;
% T2=A1*A2;
% T3=A1*A2*A3;
% T4=A1*A2*A3*A4;
% T5=A1*A2*A3*A4*A5;
T6=A1*A2*A3*A4*A5*A6;

Ox = T6(1,4);
Oy = T6(2,4);
Oz = T6(3,4);
p=[Ox;Oy;Oz]

R=T6(1:3,1:3)

== matlab function Unity_6DOFMICO_Inversekine_v8/Trajectory Planning/Iterator/Subsystem/MATLAB Function ==
  data: x output; u input; y output; z output
function [x,y,z] = fcn(u)
if u==1   %+x
    x=0.01;y=0;z=0;
elseif u==2  %-x
    x=-0.01;y=0;z=0;
elseif u==3   %+y
    x=0;y=0.01;z=0;
elseif u==4   %-y
    x=0;y=-0.01;z=0;
elseif u==5   %+z
    x=0;y=0;z=0.01;
elseif u==6    %-z
    x=0;y=0;z=-0.01;
else u==7
    x=0;y=0;z=0;
end
end
